simulink model "Sistema_realimentado"  (R2014a)
settings: Solver=ode45  StartTime=0.0  StopTime=10.0  RelTol=1e-3
values from neighbouring files (symbols this model uses):
  b = 1.1    [TP1.m]
  J = 15    [TP1.m]
  K = 6.7628    [TP1.m]
  L = 2.886e-3    (= 0.002886)    [TP1.m]
  R = 50.296e-3    (= 0.050296)    [TP1.m]
libraries: cstblocks x1
settings Model: Creator=lraff  LastModifiedBy=lraff

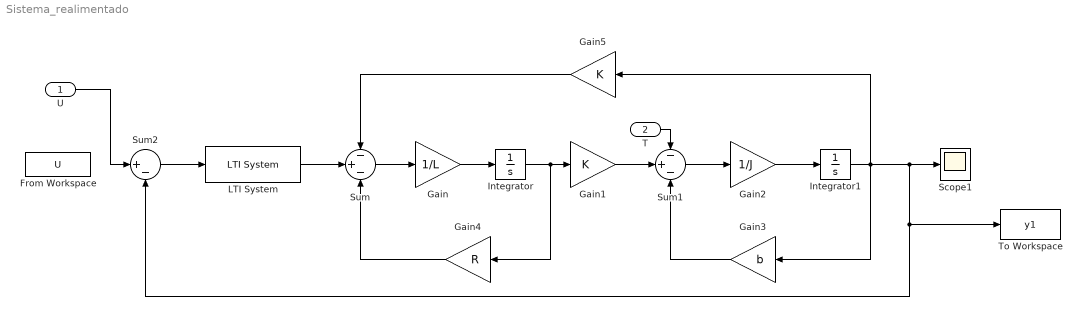
== system Sistema_realimentado ==
  U : Inport
  T : Inport  Port=2
  From Workspace : FromWorkspace  VariableName=U  SampleTime=0
  Gain : Gain  Gain=1/L
  Gain1 : Gain  Gain=K
  Gain2 : Gain  Gain=1/J
  Gain3 : Gain  Gain=b
  Gain4 : Gain  Gain=R
  Gain5 : Gain  Gain=K
  Integrator : Integrator
  Integrator1 : Integrator
  LTI System : cstblocks/LTI System  sys=C  IC=[]
  Scope1 : Scope
  Sum : Sum  Inputs=-+-
  Sum1 : Sum  Inputs=-+-
  Sum2 : Sum  Inputs=|+-
  To Workspace : ToWorkspace  VariableName=y1  SaveFormat=Timeseries  SampleTime=-1
  wires:
  Sum/1 -> Gain/1
  Gain/1 -> Integrator/1
  Integrator/1 -> Gain4/1, Gain1/1
  Gain1/1 -> Sum1/2
  Sum1/1 -> Gain2/1
  Gain2/1 -> Integrator1/1
  Gain3/1 -> Sum1/3
  Gain4/1 -> Sum/3
  Gain5/1 -> Sum/1
  LTI System/1 -> Sum/2
  Sum2/1 -> LTI System/1
  Integrator1/1 -> To Workspace/1, Sum2/2, Scope1/1, Gain5/1, Gain3/1
  U/1 -> Sum2/1
  T/1 -> Sum1/1
